simulink library "Springs_Axle2_Independent"  (R2025a)
settings: Solver=VariableStepAuto  StartTime=0.0  StopTime=10.0  RelTol=1e-3
libraries: fl_lib x4, Spring_Element x4
Description:
  | Component of Simscape Vehicle Templates Library
  | 
  | Copyright 2018-2025 The MathWorks, Inc.
settings Model: Creator=smiller  LastModifiedBy=smiller
settings SolverCC: AlgebraicLoopSolver=TrustRegion
settings DataIOCC: ReturnWorkspaceOutputs=off
settings OptimizationCC: ReuseModelBlockBuffer=off
settings DebuggingCC: UnconnectedInputMsg=warning  UnconnectedOutputMsg=warning  UnconnectedLineMsg=warning  ArithmeticOperatorsInVariantConditions=warning
settings ModelReferenceCC: EnableRefExpFcnMdlSchedulingChecks=on
settings SFSimCC: CustomCodeUndefinedFunction=UseInterfaceOnly
settings RTWCC: GPUComputeCapability=3.5  DLArmComputeVersion=19.05

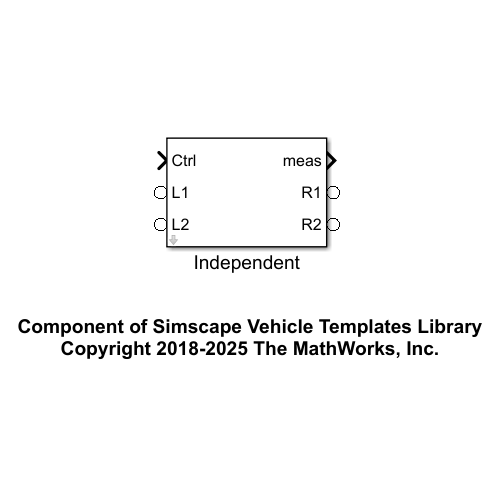
[thumbnail: Simulink's stored preview of the top-level diagram]
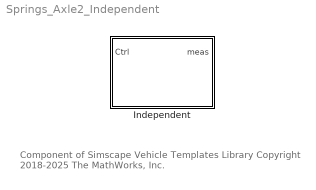
== system Springs_Axle2_Independent ==
  note: Component of Simscape Vehicle Templates Library
      | Copyright 2018-2025 The MathWorks, Inc.
  Independent : Subsystem  VariantControl=Independent  mask(Independent Springs){}
      mask help: Models independent left and right springs on two axles

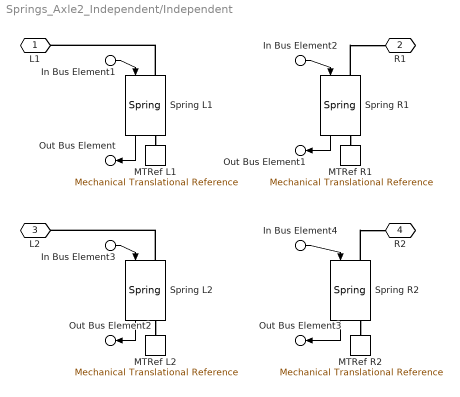
== system Springs_Axle2_Independent/Independent ==
  In Bus Element1 : Inport  PortName=Ctrl  Element=L1
  In Bus Element2 : Inport  PortName=Ctrl  Element=R1
  In Bus Element3 : Inport  PortName=Ctrl  Element=L2
  In Bus Element4 : Inport  PortName=Ctrl  Element=R2
  MTRef L1 : fl_lib/Mechanical/Translational Elements/Mechanical Translational Reference
  MTRef L2 : fl_lib/Mechanical/Translational Elements/Mechanical Translational Reference
  MTRef R1 : fl_lib/Mechanical/Translational Elements/Mechanical Translational Reference
  MTRef R2 : fl_lib/Mechanical/Translational Elements/Mechanical Translational Reference
  Spring L1 : Spring_Element/Spring  VariantControl=Variant1  LabelModeActiveChoice=Linear  Spring=Spring.Axle1  VariantLabel=Spring.Axle1.class.Value
      settings: AttributesFormatString=%<ActiveVariant>
  Spring L2 : Spring_Element/Spring  VariantControl=Variant1  LabelModeActiveChoice=Linear  Spring=Spring.Axle2  VariantLabel=Spring.Axle2.class.Value
      settings: AttributesFormatString=%<ActiveVariant>
  Spring R1 : Spring_Element/Spring  VariantControl=Variant1  LabelModeActiveChoice=Linear  Spring=Spring.Axle1  VariantLabel=Spring.Axle1.class.Value
      settings: AttributesFormatString=%<ActiveVariant>
  Spring R2 : Spring_Element/Spring  VariantControl=Variant1  LabelModeActiveChoice=Linear  Spring=Spring.Axle2  VariantLabel=Spring.Axle2.class.Value
      settings: AttributesFormatString=%<ActiveVariant>
  L1 : PMIOPort  Side=Left
  R1 : PMIOPort  Port=2  Side=Right
  L2 : PMIOPort  Port=3  Side=Left
  R2 : PMIOPort  Port=4  Side=Right
  Out Bus Element : Outport  VectorParamsAs1DForOutWhenUnconnected=off  PortName=meas  Element=L1
  Out Bus Element1 : Outport  VectorParamsAs1DForOutWhenUnconnected=off  PortName=meas  Element=R1
  Out Bus Element2 : Outport  VectorParamsAs1DForOutWhenUnconnected=off  PortName=meas  Element=L2
  Out Bus Element3 : Outport  VectorParamsAs1DForOutWhenUnconnected=off  PortName=meas  Element=R2
  wires:
  Spring R2/1 -> Out Bus Element3/1
  In Bus Element4/1 -> Spring R2/1
  Spring L2/1 -> Out Bus Element2/1
  In Bus Element3/1 -> Spring L2/1
  Spring R1/1 -> Out Bus Element1/1
  In Bus Element2/1 -> Spring R1/1
  Spring L1/1 -> Out Bus Element/1
  In Bus Element1/1 -> Spring L1/1
  connections:
  Spring L1/RConn1 -- MTRef L1/LConn1
  Spring L1/LConn1 -- L1/RConn1
  Spring L2/RConn1 -- MTRef L2/LConn1
  Spring L2/LConn1 -- L2/RConn1
  Spring R2/RConn1 -- MTRef R2/LConn1
  Spring R2/LConn1 -- R2/RConn1
  Spring R1/RConn1 -- MTRef R1/LConn1
  Spring R1/LConn1 -- R1/RConn1
